simulink model "RW_Simulink_Controller"  (R2017b)
settings: Solver=VariableStepAuto  StartTime=0  StopTime=20  FixedStep=0.001  MaxStep=1e-4  MinStep=1e-5  RelTol=1e-4
values from neighbouring files (symbols this model uses):
  b = 1.144e-08    [RW_Controller.m]
  d = 9.94e-10    [RW_Controller.m]
  l = 0.23    [RW_Controller.m]
settings Model: Creator=Nicky  LastModifiedBy=Nicky
settings SolverCC: ZeroCrossAlgorithm=Adaptive  AlgebraicLoopSolver=LineSearch  AutoInsertRateTranBlk=on
settings DebuggingCC: MaxConsecutiveZCsMsg=none
settings CodeAppCC: StateflowObjectComments=on
settings SimscapeCC: SimscapeNormalizeSystem=off

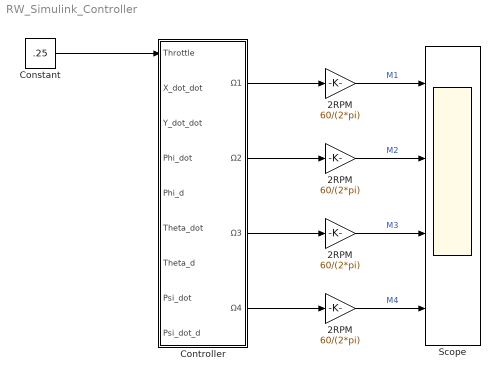
== system RW_Simulink_Controller ==
  2RPM : Gain  Gain=60/(2*pi)
  "2RPM " : Gain  Gain=60/(2*pi)
  "2RPM  " : Gain  Gain=60/(2*pi)
  "2RPM    " : Gain  Gain=60/(2*pi)
  Constant : Constant  Value=.25
  Controller : Subsystem
  Scope : Scope  NumInputPorts=4
  wires:
  Controller/1(Ω1) -> 2RPM/1
  Controller/2(Ω2) -> "2RPM "/1
  Controller/3(Ω3) -> "2RPM  "/1
  Controller/4(Ω4) -> "2RPM    "/1
  2RPM/1 -> Scope/1  "M1"
  "2RPM "/1 -> Scope/2  "M2"
  "2RPM  "/1 -> Scope/3  "M3"
  "2RPM    "/1 -> Scope/4  "M4"
  Constant/1 -> Controller/1(Throttle)

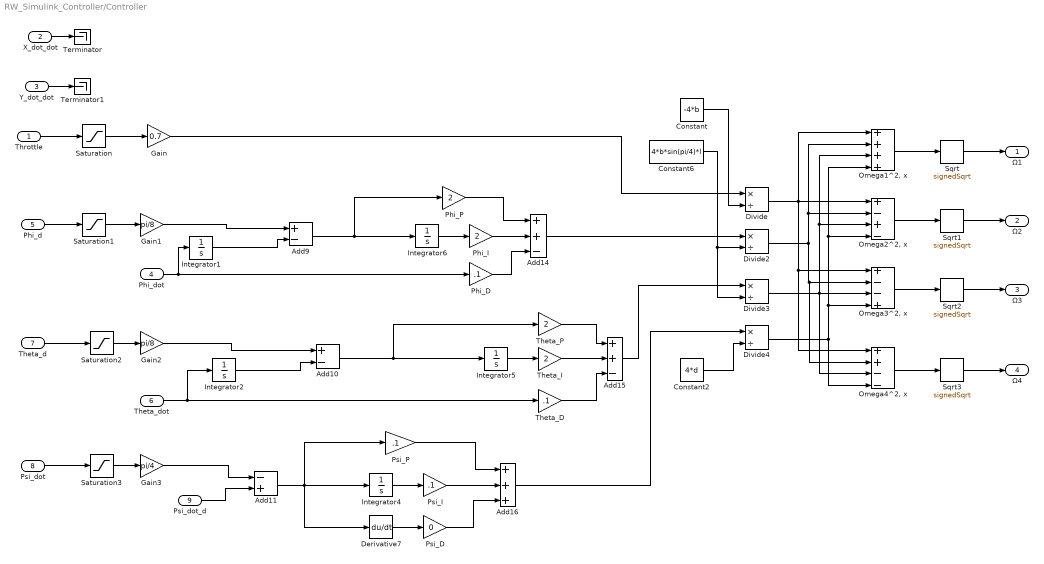
== system RW_Simulink_Controller/Controller ==
  Throttle : Inport
  X_dot_dot : Inport  Port=2
  Y_dot_dot : Inport  Port=3
  Phi_dot : Inport  Port=4
  Phi_d : Inport  Port=5
  Theta_dot : Inport  Port=6
  Theta_d : Inport  Port=7
  Psi_dot : Inport  Port=8
  Psi_dot_d : Inport  Port=9
  Add10 : Sum  Inputs=+-
  Add11 : Sum  Inputs=-+
  Add14 : Sum  Inputs=++-
  Add15 : Sum  Inputs=++-
  Add16 : Sum  Inputs=+++
  Add9 : Sum  Inputs=+-
  Constant : Constant  Value=-4*b
  Constant2 : Constant  Value=4*d
  Constant6 : Constant  Value=4*b*sin(pi/4)*l
  Derivative7 : Derivative
  Divide{,2..4} (4 alike) : Product  Inputs=*/
  Gain : Gain  Gain=0.7
  Gain1 : Gain  Gain=pi/8
  Gain2 : Gain  Gain=pi/8
  Gain3 : Gain  Gain=pi/4
  Integrator1 : Integrator  WrapState=on
  Integrator2 : Integrator  WrapState=on
  Integrator4 : Integrator
  Integrator5 : Integrator
  Integrator6 : Integrator
  "Omega1^2, x" : Sum  Inputs=++++
  "Omega2^2, x" : Sum  Inputs=+-+-
  "Omega3^2, x" : Sum  Inputs=+--+
  "Omega4^2, x" : Sum  Inputs=++--
  Phi_D : Gain  Gain=.1
  Phi_I : Gain  Gain=2
  Phi_P : Gain  Gain=2
  Psi_D : Gain  Gain=0
  Psi_I : Gain  Gain=.1
  Psi_P : Gain  Gain=.1
  Saturation : Saturate  UpperLimit=1  LowerLimit=0
  Saturation1 : Saturate  UpperLimit=1  LowerLimit=-1
  Saturation2 : Saturate  UpperLimit=1  LowerLimit=-1
  Saturation3 : Saturate  UpperLimit=1  LowerLimit=-1
  Sqrt{,1..3} (4 alike) : Sqrt  Operator=signedSqrt  SaturateOnIntegerOverflow=on
  Terminator : Terminator
  Terminator1 : Terminator
  Theta_D : Gain  Gain=.1
  Theta_I : Gain  Gain=2
  Theta_P : Gain  Gain=2
  Ω1 : Outport
  Ω2 : Outport  Port=2
  Ω3 : Outport  Port=3
  Ω4 : Outport  Port=4
  wires:
  Theta_I/1 -> Add15/2
  Throttle/1 -> Saturation/1
  Add11/1 -> Derivative7/1, Integrator4/1, Psi_P/1
  Theta_P/1 -> Add15/1
  Integrator4/1 -> Psi_I/1
  Add9/1 -> Integrator6/1, Phi_P/1
  Derivative7/1 -> Psi_D/1
  Psi_D/1 -> Add16/3
  Psi_I/1 -> Add16/2
  Integrator6/1 -> Phi_I/1
  Phi_dot/1 -> Phi_D/1, Integrator1/1
  Phi_D/1 -> Add14/3
  Theta_D/1 -> Add15/3
  Integrator5/1 -> Theta_I/1
  Add10/1 -> Theta_P/1, Integrator5/1
  Phi_I/1 -> Add14/2
  Theta_dot/1 -> Integrator2/1, Theta_D/1
  Phi_P/1 -> Add14/1
  Psi_P/1 -> Add16/1
  Constant6/1 -> Divide3/2, Divide2/2
  Add14/1 -> Divide2/1
  Add15/1 -> Divide3/1
  Gain/1 -> Divide/1
  Constant/1 -> Divide/2
  Constant2/1 -> Divide4/2
  Add16/1 -> Divide4/1
  Sqrt/1 -> Ω1/1
  Sqrt1/1 -> Ω2/1
  Sqrt2/1 -> Ω3/1
  Sqrt3/1 -> Ω4/1
  Divide4/1 -> "Omega3^2, x"/4, "Omega2^2, x"/4, "Omega1^2, x"/4, "Omega4^2, x"/4
  Divide2/1 -> "Omega4^2, x"/2, "Omega3^2, x"/2, "Omega2^2, x"/2, "Omega1^2, x"/2
  Divide3/1 -> "Omega4^2, x"/3, "Omega3^2, x"/3, "Omega2^2, x"/3, "Omega1^2, x"/3
  Divide/1 -> "Omega4^2, x"/1, "Omega3^2, x"/1, "Omega2^2, x"/1, "Omega1^2, x"/1
  "Omega1^2, x"/1 -> Sqrt/1
  "Omega2^2, x"/1 -> Sqrt1/1
  "Omega3^2, x"/1 -> Sqrt2/1
  "Omega4^2, x"/1 -> Sqrt3/1
  Phi_d/1 -> Saturation1/1
  Integrator1/1 -> Add9/2
  Integrator2/1 -> Add10/2
  Psi_dot/1 -> Saturation3/1
  Psi_dot_d/1 -> Add11/2
  Saturation/1 -> Gain/1
  Saturation1/1 -> Gain1/1
  Gain1/1 -> Add9/1
  Saturation2/1 -> Gain2/1
  Theta_d/1 -> Saturation2/1
  Gain2/1 -> Add10/1
  Saturation3/1 -> Gain3/1
  Gain3/1 -> Add11/1
  X_dot_dot/1 -> Terminator/1
  Y_dot_dot/1 -> Terminator1/1
